simulink model "sim_tutorial3"  (Simulink 3.00)
settings: Solver=ode23tb  StartTime=0.0  StopTime=1.5  RelTol=1e-2
values from neighbouring files (symbols this model uses):
  B = [bu*[Rot.Fu_cos Rot.Fu_sin] b]    [tst_sim3.m]
  c = [1 0 0]    [drawrot3dexp.m]    (also in drawrot3dmode.m)
  D = [0*d(:,1:2) d]    [tst_sim3.m]
undefined symbols (not defined in the file or in its folder): a
libraries: simulink3 x1

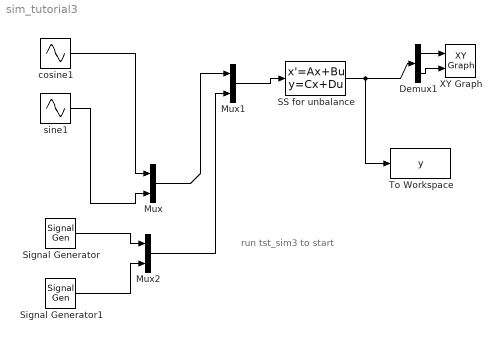
== system sim_tutorial3 ==
  note: run
      | tst_sim3
      | to start
  Demux1 : Demux  Outputs=2
  Mux : Mux  Inputs=2
  Mux1 : Mux  Inputs=2
  Mux2 : Mux  Inputs=2
  SS for unbalance : StateSpace  A=a  B=B  C=c  D=D  X0=0
  Signal Generator : SignalGenerator  WaveForm=square  Amplitude=1  Frequency=1  Units=Hertz
  Signal Generator1 : SignalGenerator  WaveForm=square  Amplitude=1  Frequency=.9  Units=Hertz
  To Workspace : ToWorkspace  VariableName=y  SampleTime=-1  SaveFormat=StructureWithTime
  XY Graph : simulink3/Sinks/XY Graph  xmin=-3e-6  xmax=3e-6  ymin=-3e-6  ymax=3e-6  st=-1
  cosine1 : Sin  Amplitude=1  Frequency=1.21  Phase=pi/2  SampleTime=0
  sine1 : Sin  Amplitude=1  Frequency=1  Phase=0  SampleTime=0
  wires:
  Demux1/2 -> XY Graph/2
  Demux1/1 -> XY Graph/1
  sine1/1 -> Mux/2
  cosine1/1 -> Mux/1
  Mux1/1 -> SS for unbalance/1
  Mux/1 -> Mux1/1
  Signal Generator/1 -> Mux2/1
  Signal Generator1/1 -> Mux2/2
  Mux2/1 -> Mux1/2
  SS for unbalance/1 -> Demux1/1, To Workspace/1
